simulink model "AGC30Model_ex1_11"  (R2021a)
settings: Solver=ode4  StartTime=stime  StopTime=etime  FixedStep=dtload  RelTol=1e-3
values from neighbouring files (symbols this model uses):
  AL_A = 0.3    [init_lfc_model.m]
  AL_B = 0.3    [init_lfc_model.m]
  DELTA_CC = Delta_cc_ty(TY_CC)    [load_thermal_constants.m]
  DELTA_ST = Delta_st_ty(TY_ST)    [load_thermal_constants.m]
  dtload = 0.1    [initset_dataload.m]
  F0 = 60    [init_inertia_model.m]    (also in initset_inertia.m)
  FFCS0_CC = (WF0_CC-WF_MIN_CC)./(1.0-WF_MIN_CC)    [calc_thermal_init_values.m]    (also in init_thermals.m)
  FGT_CC = Fgt_cc_ty(TY_CC)    [load_thermal_constants.m]
  FX_FB_CC = Fx_fb_cc_ty(:,TY_CC)    [load_thermal_constants.m]
  FX_FB_ST = Fx_fb_st_ty(:,TY_ST)    [load_thermal_constants.m]
  FX_FB_WT = FX_FB_WT_ty(:,TY_WT)    [load_const_hydro_constants.m]
  FX_N_GN_VA = FX_N_GN_VA_ty(:,TY_VA)    [load_var_hydro_constants.m]
  FX_N_PM_VA = FX_N_PM_VA_ty(:,TY_VA)    [load_var_hydro_constants.m]
  FX_PTHD_ST = Fx_pthd_st_ty(:,TY_ST)    [load_thermal_constants.m]
  FX_T_PM_VA = FX_T_PM_VA_ty(:,TY_VA)    [load_var_hydro_constants.m]
  FX_TE1_CC = Fx_te1_cc_ty(:,TY_CC)    [load_thermal_constants.m]
  FX_TE2_CC = Fx_te2_cc_ty(:,TY_CC)    [load_thermal_constants.m]
  FX_Y_GN_VA = FX_Y_GN_VA_ty(:,TY_VA)    [load_var_hydro_constants.m]
  FX_Y_PM_VA = FX_Y_PM_VA_ty(:,TY_VA)    [load_var_hydro_constants.m]
  FY_FB_CC = Fy_fb_cc_ty(:,TY_CC)    [load_thermal_constants.m]
  FY_FB_ST = Fy_fb_st_ty(:,TY_ST)    [load_thermal_constants.m]
  FY_FB_WT = FY_FB_WT_ty(:,TY_WT)    [load_const_hydro_constants.m]
  FY_N_GN_VA = FY_N_GN_VA_ty(:,TY_VA)    [load_var_hydro_constants.m]
  FY_N_PM_VA = FY_N_PM_VA_ty(:,TY_VA)    [load_var_hydro_constants.m]
  FY_PTHD_ST = Fy_pthd_st_ty(:,TY_ST)    [load_thermal_constants.m]
  FY_T_PM_VA = FY_T_PM_VA_ty(:,TY_VA)    [load_var_hydro_constants.m]
  FY_TE1_CC = Fy_te1_cc_ty(:,TY_CC)    [load_thermal_constants.m]
  FY_TE2_CC = Fy_te2_cc_ty(:,TY_CC)    [load_thermal_constants.m]
  FY_Y_GN_VA = FY_Y_GN_VA_ty(:,TY_VA)    [load_var_hydro_constants.m]
  FY_Y_PM_VA = FY_Y_PM_VA_ty(:,TY_VA)    [load_var_hydro_constants.m]
  G_cost = [Cost(:,3) ... (first row only)    [initset_dataload.m]
  G_down_limit = max(G_down_limit, G_out_pre - G_speed*5)    [calc_edc_output.m]    (also in edc.m; initset_dataload.m = csvread('G_down_plan_limit.csv',0,1))
  G_G_ST = G_g_st_ty(TY_ST)    [load_thermal_constants.m]
  G_speed = u(220:249,1)    [calc_edc_output.m]    (also in edc.m; initset_dataload.m = G_speed(:,1))
  GF_CC = [1, 1, 1, 1, 1,            1, 1, 1, 1, 1]    [init_thermal_model.m]
  GF_ST = [1, 1, 1, 1, 1, 1, 1,            1, 1, 1, 1,            1, 1, 1, 1, 1, 1]    [init_thermal_model.m]
  GMW_CC = Gmw_cc_ty(TY_CC)    [load_thermal_constants.m]
  GMW_ST = Gmw_st_ty(TY_ST)    [load_thermal_constants.m]
  GMW_VA = GMW_VA_ty(TY_VA)    [load_var_hydro_constants.m]
  GMW_WT = GMW_WT_ty(TY_WT)    [load_const_hydro_constants.m]
  HC_CC = Hc_cc_ty(TY_CC)    [load_thermal_constants.m]
  HT_CC = Ht_cc_ty(TY_CC)    [load_thermal_constants.m]
  IGV0_CC = WF0_CC    [calc_thermal_init_values.m]    (also in init_thermals.m)
  inertia_input = inertia_input'    [initset_dataload.m]
  K1_CONV_VA = K1_CONV_VA_ty(TY_VA)    [load_var_hydro_constants.m]
  K1_CONV_WT = K1_CONV_WT_ty(TY_WT)    [load_const_hydro_constants.m]
  K2_SERV_VA = K2_SERV_VA_ty(TY_VA)    [load_var_hydro_constants.m]
  K2_SERV_WT = K2_SERV_WT_ty(TY_WT)    [load_const_hydro_constants.m]
  K_A = 0.1    [init_lfc_model.m]
  K_B = 0.1    [init_lfc_model.m]
  K_G_ST = K_g_st_ty(TY_ST)    [load_thermal_constants.m]
  K_IGV_CC = K_igv_cc_ty(TY_CC)    [load_thermal_constants.m]
  K_L = 2.0    (= 2)    [init_inertia_model.m]    (also in initset_inertia.m)
  K_MW_GV_VA = K_MW_GV_VA_ty(TY_VA)    [load_var_hydro_constants.m]
  K_PREF_ST = K_pref_st_ty(TY_ST)    [load_thermal_constants.m]
  K_SD_VA = K_SD_VA_ty(TY_VA)    [load_var_hydro_constants.m]
  K_SD_WT = K_SD_WT_ty(TY_WT)    [load_const_hydro_constants.m]
  K_SEQ_WT = K_SEQ_WT_ty(TY_WT)    [load_const_hydro_constants.m]
  K_TE_CC = K_te_cc_ty(TY_CC)    [load_thermal_constants.m]
  KD_PID_VA = KD_PID_VA_ty(TY_VA)    [load_var_hydro_constants.m]
  KD_PID_WT = KD_PID_WT_ty(TY_WT)    [load_const_hydro_constants.m]
  KD_SG_GN_VA = KD_SG_GN_VA_ty(TY_VA)    [load_var_hydro_constants.m]
  KD_SG_PM_VA = KD_SG_PM_VA_ty(TY_VA)    [load_var_hydro_constants.m]
  KGT_CC = FGT_CC./((TFR_CC-TER_CC)-(TDR_CC-TIR_CC))    [calc_thermal_init_values.m]    (also in init_thermals.m)
  KI_PID_VA = KI_PID_VA_ty(TY_VA)    [load_var_hydro_constants.m]
  KI_PID_WT = KI_PID_WT_ty(TY_WT)    [load_const_hydro_constants.m]
  KI_SG_GN_VA = KI_SG_GN_VA_ty(TY_VA)    [load_var_hydro_constants.m]
  KI_SG_PM_VA = KI_SG_PM_VA_ty(TY_VA)    [load_var_hydro_constants.m]
  KP_A = 1.0    (= 1)    [init_lfc_model.m]
  KP_B = 1.0    (= 1)    [init_lfc_model.m]
  KP_PID_VA = KP_PID_VA_ty(TY_VA)    [load_var_hydro_constants.m]
  KP_PID_WT = KP_PID_WT_ty(TY_WT)    [load_const_hydro_constants.m]
  KP_SG_GN_VA = KP_SG_GN_VA_ty(TY_VA)    [load_var_hydro_constants.m]
  KP_SG_PM_VA = KP_SG_PM_VA_ty(TY_VA)    [load_var_hydro_constants.m]
  KST_CC = (1.0-FGT_CC)./TER_CC    [calc_thermal_init_values.m]    (also in init_thermals.m)
  L_FUEL_CC = L_fuel_cc_ty(TY_CC)    [load_thermal_constants.m]
  L_G_ST = L_g_st_ty(TY_ST)    [load_thermal_constants.m]
  L_IGV_CC = L_igv_cc_ty(TY_CC)    [load_thermal_constants.m]
  L_LL_ST = L_ll_st_ty(TY_ST)    [load_thermal_constants.m]
  L_MWD_CC = L_mwd_cc_ty(TY_CC)    [load_thermal_constants.m]
  L_MWD_GN_VA = L_MWD_GN_VA_ty(TY_VA)    [load_var_hydro_constants.m]
  L_MWD_PM_VA = L_MWD_PM_VA_ty(TY_VA)    [load_var_hydro_constants.m]
  L_MWD_ST = L_mwd_st_ty(TY_ST)    [load_thermal_constants.m]
  L_MWD_WT = L_MWD_WT_ty(TY_WT)    [load_const_hydro_constants.m]
  L_PREF_CC = L_pref_cc_ty(TY_CC)    [load_thermal_constants.m]
  L_PREF_ST = L_pref_st_ty(TY_ST)    [load_thermal_constants.m]
  LFC_cycle = 5.0    (= 5)    [init_lfc_model.m]
  load_input = load_input(:,stime+1:etime+1)    [initset_dataload.m]
  M_VA = M_VA_ty(TY_VA)    [load_var_hydro_constants.m]
  MVABase = 1000    [init_inertia_model.m]    (also in initset_inertia.m)
  MW0_ST = zeros(1,17)    [calc_thermal_init_values.m]    (also in init_thermals.m)
  MW0_WT = zeros(1,2)    [calc_const_hydro_init_values.m]    (also in init_conhydros.m)
  P_G_CONV_WT = P_G_CONV_WT_ty(TY_WT)    [load_const_hydro_constants.m]
  PG_INIT_CC = PMWD_SCHEDULE(1,19:28)'    [calc_thermal_init_values.m]    (also in init_thermals.m)
  PLM_CC = Plm_cc_ty(TY_CC)    [load_thermal_constants.m]
  PLM_ST = Plm_st_ty(TY_ST)    [load_thermal_constants.m]
  PMAX_B = 360.0    (= 360)    [init_lfc_model.m]
  PMIN_B = -360.0    (= -360)    [init_lfc_model.m]
  PMST0_CC = zeros(1, 10)    [calc_thermal_init_values.m]    (also in init_thermals.m)
  PMWD_EDC0 = zeros(1,30)    [init_edc_model.m]    (also in initset_edc.m)
  PMWD_SCHEDULE = u(3:32,1)    [calc_edc_output.m]    (also in edc.m; init_edc_model.m = g_out_input'; initset_edc.m = g_out_input')
  PRC_CC = Prc_cc_ty(TY_CC)    [load_thermal_constants.m]
  PRT_CC = PRC_CC.*(1-EP_CC)    [calc_thermal_init_values.m]    (also in init_thermals.m)
  PTH0_ST = zeros(1,17)    [calc_thermal_init_values.m]    (also in init_thermals.m)
  R_LL_ST = R_ll_st_ty(TY_ST)    [load_thermal_constants.m]
  R_MWD_CC = R_mwd_cc_ty(TY_CC)    [load_thermal_constants.m]
  R_MWD_ST = R_mwd_st_ty(TY_ST)    [load_thermal_constants.m]
  R_PREF_CC = R_pref_cc_ty(TY_CC)    [load_thermal_constants.m]
  RA_A = G_speed'    [init_lfc_model.m]
  RA_B = 96.0    (= 96)    [init_lfc_model.m]
  RATE_GN_VA = RATE_GN_VA_ty(TY_VA)    [load_var_hydro_constants.m]
  RATE_PM_VA = RATE_PM_VA_ty(TY_VA)    [load_var_hydro_constants.m]
  RC_CC = Rc_cc_ty(TY_CC)    [load_thermal_constants.m]
  RT_CC = Rt_cc_ty(TY_CC)    [load_thermal_constants.m]
  SW_T_ST = Sw_t_st_ty(TY_ST)    [load_thermal_constants.m]
  T1_B_ST = T1_b_st_ty(TY_ST)    [load_thermal_constants.m]
  T1_CONV_VA = T1_CONV_VA_ty(TY_VA)    [load_var_hydro_constants.m]
  T1_CONV_WT = T1_CONV_WT_ty(TY_WT)    [load_const_hydro_constants.m]
  T1_G_ST = T1_g_st_ty(TY_ST)    [load_thermal_constants.m]
  T2_B_ST = T2_b_st_ty(TY_ST)    [load_thermal_constants.m]
  ... (+53 more)
undefined symbols (not defined in the file or in its folder): DELTA_B, DiscIntNeverNeededParam, FX_FB_ST_OA, FX_PTHD_ST_OA, FY_FB_ST_OA, FY_PTHD_ST_OA, G_G_ST_OA, K_G_ST_OA, K_PREF_ST_OA, MW0_ST_OA, N_GN_INIT_VA, N_PM_INIT_VA, PLM_B, R_LL_ST_OA, T1_B_ST_OA, T1_G_ST_OA, T2_B_ST_OA, T2_G_ST_OA, T3_B_ST_OA, T4_G_ST_OA, T5_G_ST_OA, T_LL_ST_OA, T_PREF_ST_OA, Y_GN_INIT_VA, Y_PM_INIT_VA
libraries: simulink_extras x87, simulink x42, pid_lib x1
(part 3 of 5)

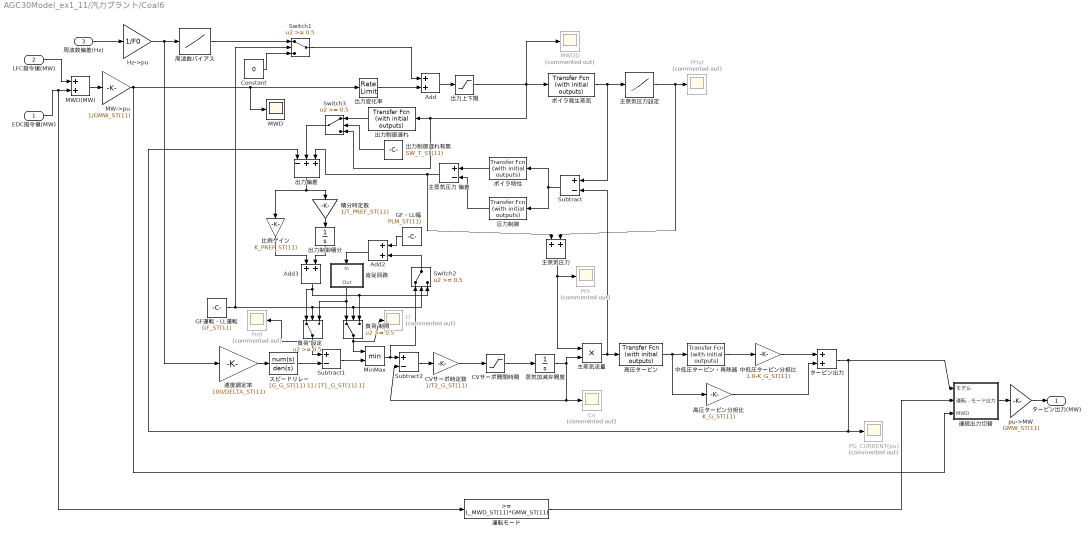
== system AGC30Model_ex1_11/汽力プラント/Coal6 ==
  EDC指令値(MW) : Inport
  LFC指令値(MW) : Inport  Port=2
  周波数偏差(Hz) : Inport  Port=3
  Add : Sum
  Add2 : Sum
  Add3 : Sum
  CVサーボ時定数 : Gain  Gain=1/T2_G_ST(11)
  CVサーボ開閉時間 : Saturate  UpperLimit=1/T3_G_ST(11)  LowerLimit=1/T6_G_ST(11)
  Constant : Constant  Value=0
  Cv : Scope  Commented=on
  GF・LL幅 : Constant  Value=PLM_ST(11)
  GF運転・LL運転 : Constant  Value=GF_ST(11)
  Hz->pu : Gain  Gain=1/F0
  Ll : Scope  Commented=on
  MW->pu : Gain  Gain=1/GMW_ST(11)
  MWD : Scope
  MWD(MW) : Sum
  MWDD : Scope  Commented=on
  MinMax : MinMax  Inputs=2
  PG_CURRENT(pu) : Scope  Commented=on
  Pref : Scope  Commented=on
  Pth : Scope  Commented=on
  Pthd : Scope  Commented=on
  Subtract : Sum  Inputs=+-
  Subtract1 : Sum  Inputs=+-
  Subtract2 : Sum  Inputs=+-
  Switch1 : Switch  Threshold=0.5
  Switch2 : Switch  Threshold=0.5
  Switch3 : Switch  Threshold=0.5
  pu->MW : Gain  Gain=GMW_ST(11)
  スピードリレー : TransferFcn  Numerator=[G_G_ST(11) 1]  Denominator=[T1_G_ST(11) 1]
  タービン出力 : Sum
  ボイラ特性 : simulink_extras/Additional Linear/Transfer Fcn (with initial outputs)  N=[1]  D=[T2_B_ST(11) 1]  Y0=0  U0=0
  ボイラ発生蒸気 : simulink_extras/Additional Linear/Transfer Fcn (with initial outputs)  N=[1]  D=[T1_B_ST(11) 1]  Y0=MW0_ST(11)  U0=MW0_ST(11)
  中低圧タービン・再熱器 : simulink_extras/Additional Linear/Transfer Fcn (with initial outputs)  N=[1]  D=[T5_G_ST(11) 1]  Y0=MW0_ST(11)  U0=MW0_ST(11)
  中低圧タービン分担比 : Gain  Gain=1.0-K_G_ST(11)
  主蒸気圧力 : Sum
  主蒸気圧力 偏差 : Sum  Inputs=+-
  主蒸気圧力設定 : Lookup  InputValues=FX_PTHD_ST(:,11)  Table=FY_PTHD_ST(:,11)  LookUpMeth=Interpolation-Use End Values
  主蒸気流量 : Product  RndMeth=Zero
  出力上下限 : Saturate  UpperLimit=U_MWD_ST(11)  LowerLimit=L_MWD_ST(11)
  出力偏差 : Sum  Inputs=-++
  出力制御積分 : Integrator  InitialCondition=MW0_ST(11)/PTH0_ST(11)  LimitOutput=on  UpperSaturationLimit=U_PREF_ST(11)  LowerSaturationLimit=L_PREF_ST(11)
  出力制御遅れ : simulink_extras/Additional Linear/Transfer Fcn (with initial outputs)  N=[1]  D=[T_T_ST(11) 1]  Y0=MW0_ST(11)  U0=MW0_ST(11)
  出力制御遅れ有無 : Constant  Value=SW_T_ST(11)
  出力変化率 : RateLimiter  RisingSlewLimit=R_MWD_ST(11)/60  FallingSlewLimit=-R_MWD_ST(11)/60  SampleTimeMode=inherited  InitialCondition=MW0_ST(11)
  周波数バイアス : Lookup  InputValues=FX_FB_ST(:,11)/F0  Table=FY_FB_ST(:,11)  LookUpMeth=Interpolation-Use End Values
  圧力制御 : simulink_extras/Additional Linear/Transfer Fcn (with initial outputs)  N=[1]  D=[T3_B_ST(11) 1]  Y0=0  U0=0
  比例ゲイン : Gain  Gain=K_PREF_ST(11)
  積分時定数 : Gain  Gain=1/T_PREF_ST(11)
  蒸気加減弁開度 : Integrator  InitialCondition=MW0_ST(11)/PTH0_ST(11)  LimitOutput=on  UpperSaturationLimit=U_G_ST(11)  LowerSaturationLimit=L_G_ST(11)
  負荷 制限 : Switch  Threshold=0.5
  負荷 設定 : Switch  Threshold=0.5
  追従回路 : Subsystem
  速度調定率 : Gain  Gain=100/DELTA_ST(11)
  連続出力切替 : Subsystem
  運転モード : simulink/Logic and Bit Operations/Compare To Constant  relop=>=  const=L_MWD_ST(11)*GMW_ST(11)  OutDataTypeStr=boolean
  高圧タービン : simulink_extras/Additional Linear/Transfer Fcn (with initial outputs)  N=[1]  D=[T4_G_ST(11) 1]  Y0=MW0_ST(11)  U0=MW0_ST(11)
  高圧タービン分担比 : Gain  Gain=K_G_ST(11)
  タービン出力(MW) : Outport  VectorParamsAs1DForOutWhenUnconnected=off
  wires:
  MWD(MW)/1 -> MW->pu/1
  周波数偏差(Hz)/1 -> Hz->pu/1
  Add/1 -> 出力上下限/1
  出力変化率/1 -> Add/2
  ボイラ発生蒸気/1 -> Subtract/1, 主蒸気圧力設定/1
  出力偏差/1 -> 比例ゲイン/1, 積分時定数/1
  比例ゲイン/1 -> Add3/1
  Add3/1 -> 負荷 制限/3, Switch2/3, 負荷 設定/1
  主蒸気圧力 偏差/1 -> 主蒸気圧力/1, 出力偏差/3
  主蒸気圧力設定/1 -> Pthd/1, 主蒸気圧力/2
  主蒸気流量/1 -> Subtract/2, 高圧タービン/1
  積分時定数/1 -> 出力制御積分/1
  出力制御積分/1 -> Add3/2
  速度調定率/1 -> スピードリレー/1
  Subtract1/1 -> MinMax/2
  主蒸気圧力/1 -> 主蒸気流量/1, Pth/1
  スピードリレー/1 -> Subtract1/2
  MinMax/1 -> Subtract2/1, Switch2/1
  Subtract2/1 -> CVサーボ時定数/1
  CVサーボ時定数/1 -> CVサーボ開閉時間/1
  CVサーボ開閉時間/1 -> 蒸気加減弁開度/1
  蒸気加減弁開度/1 -> 主蒸気流量/2, Subtract2/2, Cv/1
  高圧タービン/1 -> 中低圧タービン・再熱器/1, 高圧タービン分担比/1
  中低圧タービン・再熱器/1 -> 中低圧タービン分担比/1
  高圧タービン分担比/1 -> タービン出力/2
  中低圧タービン分担比/1 -> タービン出力/1
  タービン出力/1 -> 出力偏差/1, PG_CURRENT(pu)/1, 連続出力切替/1(モデル)
  GF・LL幅/1 -> Add2/1
  Add2/1 -> 追従回路/1(In)
  ボイラ特性/1 -> 主蒸気圧力 偏差/1
  圧力制御/1 -> 主蒸気圧力 偏差/2
  Subtract/1 -> ボイラ特性/1, 圧力制御/1
  出力上下限/1 -> ボイラ発生蒸気/1, MWDD/1, 出力制御遅れ/1, Switch3/3
  GF運転・LL運転/1 -> 負荷 設定/2, 負荷 制限/2, Switch2/2, Switch1/2
  負荷 設定/1 -> Subtract1/1, Pref/1
  追従回路/1(Out) -> 負荷 制限/1, 負荷 設定/3
  Switch2/1 -> Add2/2
  MW->pu/1 -> MWD/1, 出力変化率/1, 連続出力切替/3(MWD)
  Hz->pu/1 -> 速度調定率/1, 周波数バイアス/1
  連続出力切替/1(出力) -> pu->MW/1
  pu->MW/1 -> タービン出力(MW)/1
  負荷 制限/1 -> MinMax/1, Ll/1
  周波数バイアス/1 -> Switch1/1
  Constant/1 -> Switch1/3
  Switch1/1 -> Add/1
  出力制御遅れ/1 -> Switch3/1
  Switch3/1 -> 出力偏差/2
  出力制御遅れ有無/1 -> Switch3/2
  EDC指令値(MW)/1 -> MWD(MW)/2, 運転モード/1
  LFC指令値(MW)/1 -> MWD(MW)/1
  運転モード/1 -> 連続出力切替/2(運転モード)

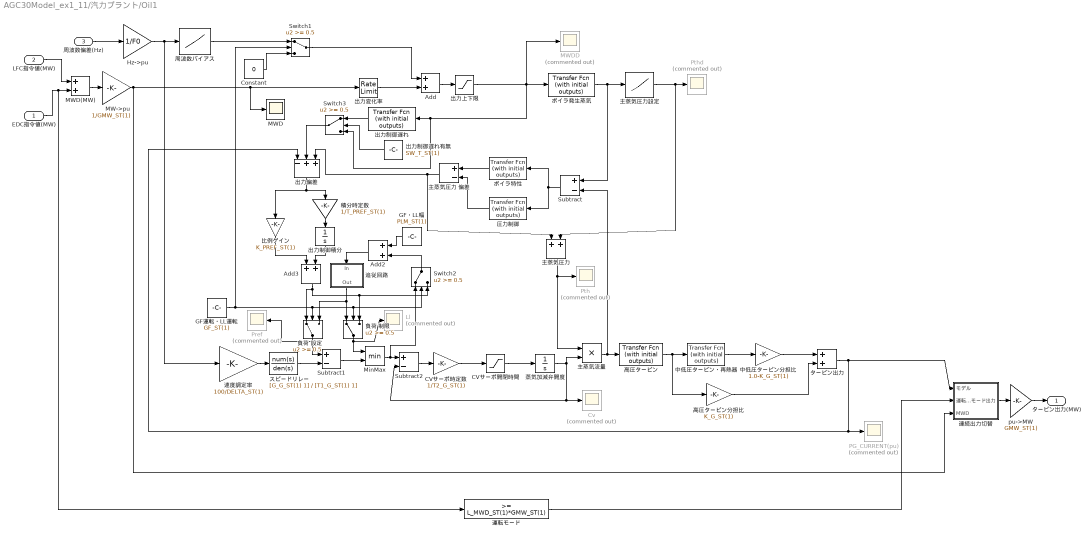
== system AGC30Model_ex1_11/汽力プラント/Oil1 ==
  EDC指令値(MW) : Inport
  LFC指令値(MW) : Inport  Port=2
  周波数偏差(Hz) : Inport  Port=3
  Add : Sum
  Add2 : Sum
  Add3 : Sum
  CVサーボ時定数 : Gain  Gain=1/T2_G_ST(1)
  CVサーボ開閉時間 : Saturate  UpperLimit=1/T3_G_ST(1)  LowerLimit=1/T6_G_ST(1)
  Constant : Constant  Value=0
  Cv : Scope  Commented=on
  GF・LL幅 : Constant  Value=PLM_ST(1)
  GF運転・LL運転 : Constant  Value=GF_ST(1)
  Hz->pu : Gain  Gain=1/F0
  Ll : Scope  Commented=on
  MW->pu : Gain  Gain=1/GMW_ST(1)
  MWD : Scope
  MWD(MW) : Sum
  MWDD : Scope  Commented=on
  MinMax : MinMax  Inputs=2
  PG_CURRENT(pu) : Scope  Commented=on
  Pref : Scope  Commented=on
  Pth : Scope  Commented=on
  Pthd : Scope  Commented=on
  Subtract : Sum  Inputs=+-
  Subtract1 : Sum  Inputs=+-
  Subtract2 : Sum  Inputs=+-
  Switch1 : Switch  Threshold=0.5
  Switch2 : Switch  Threshold=0.5
  Switch3 : Switch  Threshold=0.5
  pu->MW : Gain  Gain=GMW_ST(1)
  スピードリレー : TransferFcn  Numerator=[G_G_ST(1) 1]  Denominator=[T1_G_ST(1) 1]
  タービン出力 : Sum
  ボイラ特性 : simulink_extras/Additional Linear/Transfer Fcn (with initial outputs)  N=[1]  D=[T2_B_ST(1) 1]  Y0=0  U0=0
  ボイラ発生蒸気 : simulink_extras/Additional Linear/Transfer Fcn (with initial outputs)  N=[1]  D=[T1_B_ST(1) 1]  Y0=MW0_ST(1)  U0=MW0_ST(1)
  中低圧タービン・再熱器 : simulink_extras/Additional Linear/Transfer Fcn (with initial outputs)  N=[1]  D=[T5_G_ST(1) 1]  Y0=MW0_ST(1)  U0=MW0_ST(1)
  中低圧タービン分担比 : Gain  Gain=1.0-K_G_ST(1)
  主蒸気圧力 : Sum
  主蒸気圧力 偏差 : Sum  Inputs=+-
  主蒸気圧力設定 : Lookup  InputValues=FX_PTHD_ST(:,1)  Table=FY_PTHD_ST(:,1)  LookUpMeth=Interpolation-Use End Values
  主蒸気流量 : Product  RndMeth=Zero
  出力上下限 : Saturate  UpperLimit=U_MWD_ST(1)  LowerLimit=L_MWD_ST(1)
  出力偏差 : Sum  Inputs=-++
  出力制御積分 : Integrator  InitialCondition=MW0_ST(1)/PTH0_ST(1)  LimitOutput=on  UpperSaturationLimit=U_PREF_ST(1)  LowerSaturationLimit=L_PREF_ST(1)
  出力制御遅れ : simulink_extras/Additional Linear/Transfer Fcn (with initial outputs)  N=[1]  D=[T_T_ST(1) 1]  Y0=MW0_ST(1)  U0=MW0_ST(1)
  出力制御遅れ有無 : Constant  Value=SW_T_ST(1)
  出力変化率 : RateLimiter  RisingSlewLimit=R_MWD_ST(1)/60  FallingSlewLimit=-R_MWD_ST(1)/60  SampleTimeMode=inherited  InitialCondition=MW0_ST(1)
  周波数バイアス : Lookup  InputValues=FX_FB_ST(:,1)/F0  Table=FY_FB_ST(:,1)  LookUpMeth=Interpolation-Use End Values
  圧力制御 : simulink_extras/Additional Linear/Transfer Fcn (with initial outputs)  N=[1]  D=[T3_B_ST(1) 1]  Y0=0  U0=0
  比例ゲイン : Gain  Gain=K_PREF_ST(1)
  積分時定数 : Gain  Gain=1/T_PREF_ST(1)
  蒸気加減弁開度 : Integrator  InitialCondition=MW0_ST(1)/PTH0_ST(1)  LimitOutput=on  UpperSaturationLimit=U_G_ST(1)  LowerSaturationLimit=L_G_ST(1)
  負荷 制限 : Switch  Threshold=0.5
  負荷 設定 : Switch  Threshold=0.5
  追従回路 : Subsystem
  速度調定率 : Gain  Gain=100/DELTA_ST(1)
  連続出力切替 : Subsystem
  運転モード : simulink/Logic and Bit Operations/Compare To Constant  relop=>=  const=L_MWD_ST(1)*GMW_ST(1)  OutDataTypeStr=boolean
  高圧タービン : simulink_extras/Additional Linear/Transfer Fcn (with initial outputs)  N=[1]  D=[T4_G_ST(1) 1]  Y0=MW0_ST(1)  U0=MW0_ST(1)
  高圧タービン分担比 : Gain  Gain=K_G_ST(1)
  タービン出力(MW) : Outport  VectorParamsAs1DForOutWhenUnconnected=off
  wires:
  MWD(MW)/1 -> MW->pu/1
  周波数偏差(Hz)/1 -> Hz->pu/1
  Add/1 -> 出力上下限/1
  出力変化率/1 -> Add/2
  ボイラ発生蒸気/1 -> Subtract/1, 主蒸気圧力設定/1
  出力偏差/1 -> 比例ゲイン/1, 積分時定数/1
  比例ゲイン/1 -> Add3/1
  Add3/1 -> 負荷 制限/3, Switch2/3, 負荷 設定/1
  主蒸気圧力 偏差/1 -> 主蒸気圧力/1, 出力偏差/3
  主蒸気圧力設定/1 -> Pthd/1, 主蒸気圧力/2
  主蒸気流量/1 -> Subtract/2, 高圧タービン/1
  積分時定数/1 -> 出力制御積分/1
  出力制御積分/1 -> Add3/2
  速度調定率/1 -> スピードリレー/1
  Subtract1/1 -> MinMax/2
  主蒸気圧力/1 -> 主蒸気流量/1, Pth/1
  スピードリレー/1 -> Subtract1/2
  MinMax/1 -> Subtract2/1, Switch2/1
  Subtract2/1 -> CVサーボ時定数/1
  CVサーボ時定数/1 -> CVサーボ開閉時間/1
  CVサーボ開閉時間/1 -> 蒸気加減弁開度/1
  蒸気加減弁開度/1 -> 主蒸気流量/2, Subtract2/2, Cv/1
  高圧タービン/1 -> 中低圧タービン・再熱器/1, 高圧タービン分担比/1
  中低圧タービン・再熱器/1 -> 中低圧タービン分担比/1
  高圧タービン分担比/1 -> タービン出力/2
  中低圧タービン分担比/1 -> タービン出力/1
  タービン出力/1 -> 出力偏差/1, PG_CURRENT(pu)/1, 連続出力切替/1(モデル)
  GF・LL幅/1 -> Add2/1
  Add2/1 -> 追従回路/1(In)
  ボイラ特性/1 -> 主蒸気圧力 偏差/1
  圧力制御/1 -> 主蒸気圧力 偏差/2
  Subtract/1 -> ボイラ特性/1, 圧力制御/1
  出力上下限/1 -> ボイラ発生蒸気/1, MWDD/1, 出力制御遅れ/1, Switch3/3
  GF運転・LL運転/1 -> 負荷 設定/2, 負荷 制限/2, Switch2/2, Switch1/2
  負荷 設定/1 -> Subtract1/1, Pref/1
  追従回路/1(Out) -> 負荷 制限/1, 負荷 設定/3
  Switch2/1 -> Add2/2
  MW->pu/1 -> MWD/1, 出力変化率/1, 連続出力切替/3(MWD)
  Hz->pu/1 -> 速度調定率/1, 周波数バイアス/1
  連続出力切替/1(出力) -> pu->MW/1
  pu->MW/1 -> タービン出力(MW)/1
  負荷 制限/1 -> MinMax/1, Ll/1
  周波数バイアス/1 -> Switch1/1
  Constant/1 -> Switch1/3
  Switch1/1 -> Add/1
  出力制御遅れ/1 -> Switch3/1
  Switch3/1 -> 出力偏差/2
  出力制御遅れ有無/1 -> Switch3/2
  EDC指令値(MW)/1 -> MWD(MW)/2, 運転モード/1
  LFC指令値(MW)/1 -> MWD(MW)/1
  運転モード/1 -> 連続出力切替/2(運転モード)

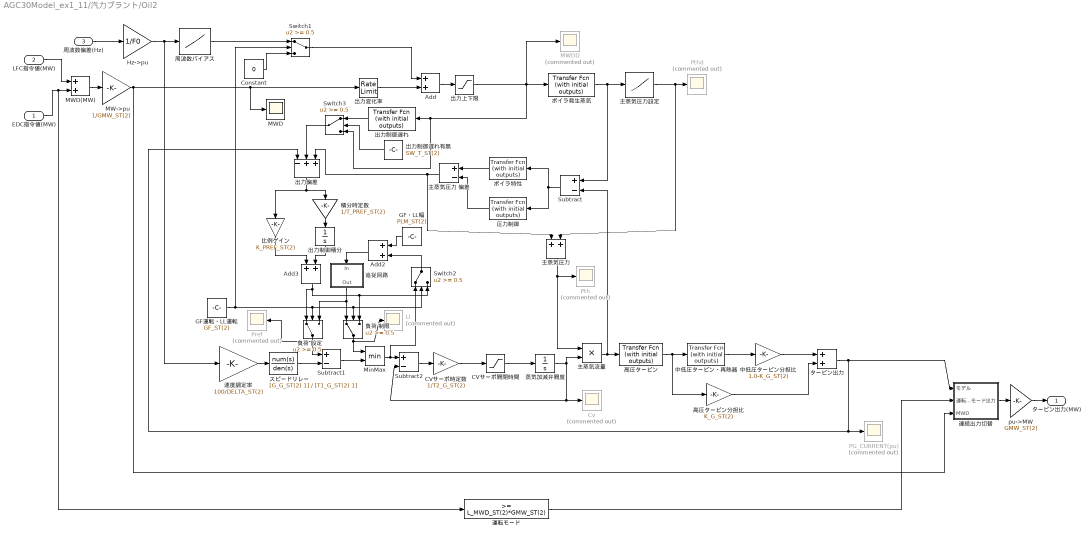
== system AGC30Model_ex1_11/汽力プラント/Oil2 ==
  EDC指令値(MW) : Inport
  LFC指令値(MW) : Inport  Port=2
  周波数偏差(Hz) : Inport  Port=3
  Add : Sum
  Add2 : Sum
  Add3 : Sum
  CVサーボ時定数 : Gain  Gain=1/T2_G_ST(2)
  CVサーボ開閉時間 : Saturate  UpperLimit=1/T3_G_ST(2)  LowerLimit=1/T6_G_ST(2)
  Constant : Constant  Value=0
  Cv : Scope  Commented=on
  GF・LL幅 : Constant  Value=PLM_ST(2)
  GF運転・LL運転 : Constant  Value=GF_ST(2)
  Hz->pu : Gain  Gain=1/F0
  Ll : Scope  Commented=on
  MW->pu : Gain  Gain=1/GMW_ST(2)
  MWD : Scope
  MWD(MW) : Sum
  MWDD : Scope  Commented=on
  MinMax : MinMax  Inputs=2
  PG_CURRENT(pu) : Scope  Commented=on
  Pref : Scope  Commented=on
  Pth : Scope  Commented=on
  Pthd : Scope  Commented=on
  Subtract : Sum  Inputs=+-
  Subtract1 : Sum  Inputs=+-
  Subtract2 : Sum  Inputs=+-
  Switch1 : Switch  Threshold=0.5
  Switch2 : Switch  Threshold=0.5
  Switch3 : Switch  Threshold=0.5
  pu->MW : Gain  Gain=GMW_ST(2)
  スピードリレー : TransferFcn  Numerator=[G_G_ST(2) 1]  Denominator=[T1_G_ST(2) 1]
  タービン出力 : Sum
  ボイラ特性 : simulink_extras/Additional Linear/Transfer Fcn (with initial outputs)  N=[1]  D=[T2_B_ST(2) 1]  Y0=0  U0=0
  ボイラ発生蒸気 : simulink_extras/Additional Linear/Transfer Fcn (with initial outputs)  N=[1]  D=[T1_B_ST(2) 1]  Y0=MW0_ST(2)  U0=MW0_ST(2)
  中低圧タービン・再熱器 : simulink_extras/Additional Linear/Transfer Fcn (with initial outputs)  N=[1]  D=[T5_G_ST(2) 1]  Y0=MW0_ST(2)  U0=MW0_ST(2)
  中低圧タービン分担比 : Gain  Gain=1.0-K_G_ST(2)
  主蒸気圧力 : Sum
  主蒸気圧力 偏差 : Sum  Inputs=+-
  主蒸気圧力設定 : Lookup  InputValues=FX_PTHD_ST(:,2)  Table=FY_PTHD_ST(:,2)  LookUpMeth=Interpolation-Use End Values
  主蒸気流量 : Product  RndMeth=Zero
  出力上下限 : Saturate  UpperLimit=U_MWD_ST(2)  LowerLimit=L_MWD_ST(2)
  出力偏差 : Sum  Inputs=-++
  出力制御積分 : Integrator  InitialCondition=MW0_ST(2)/PTH0_ST(2)  LimitOutput=on  UpperSaturationLimit=U_PREF_ST(2)  LowerSaturationLimit=L_PREF_ST(2)
  出力制御遅れ : simulink_extras/Additional Linear/Transfer Fcn (with initial outputs)  N=[1]  D=[T_T_ST(2) 1]  Y0=MW0_ST(2)  U0=MW0_ST(2)
  出力制御遅れ有無 : Constant  Value=SW_T_ST(2)
  出力変化率 : RateLimiter  RisingSlewLimit=R_MWD_ST(2)/60  FallingSlewLimit=-R_MWD_ST(2)/60  SampleTimeMode=inherited  InitialCondition=MW0_ST(2)
  周波数バイアス : Lookup  InputValues=FX_FB_ST(:,2)/F0  Table=FY_FB_ST(:,2)  LookUpMeth=Interpolation-Use End Values
  圧力制御 : simulink_extras/Additional Linear/Transfer Fcn (with initial outputs)  N=[1]  D=[T3_B_ST(2) 1]  Y0=0  U0=0
  比例ゲイン : Gain  Gain=K_PREF_ST(2)
  積分時定数 : Gain  Gain=1/T_PREF_ST(2)
  蒸気加減弁開度 : Integrator  InitialCondition=MW0_ST(2)/PTH0_ST(2)  LimitOutput=on  UpperSaturationLimit=U_G_ST(2)  LowerSaturationLimit=L_G_ST(2)
  負荷 制限 : Switch  Threshold=0.5
  負荷 設定 : Switch  Threshold=0.5
  追従回路 : Subsystem
  速度調定率 : Gain  Gain=100/DELTA_ST(2)
  連続出力切替 : Subsystem
  運転モード : simulink/Logic and Bit Operations/Compare To Constant  relop=>=  const=L_MWD_ST(2)*GMW_ST(2)  OutDataTypeStr=boolean
  高圧タービン : simulink_extras/Additional Linear/Transfer Fcn (with initial outputs)  N=[1]  D=[T4_G_ST(2) 1]  Y0=MW0_ST(2)  U0=MW0_ST(2)
  高圧タービン分担比 : Gain  Gain=K_G_ST(2)
  タービン出力(MW) : Outport  VectorParamsAs1DForOutWhenUnconnected=off
  wires:
  MWD(MW)/1 -> MW->pu/1
  周波数偏差(Hz)/1 -> Hz->pu/1
  Add/1 -> 出力上下限/1
  出力変化率/1 -> Add/2
  ボイラ発生蒸気/1 -> Subtract/1, 主蒸気圧力設定/1
  出力偏差/1 -> 比例ゲイン/1, 積分時定数/1
  比例ゲイン/1 -> Add3/1
  Add3/1 -> 負荷 制限/3, Switch2/3, 負荷 設定/1
  主蒸気圧力 偏差/1 -> 主蒸気圧力/1, 出力偏差/3
  主蒸気圧力設定/1 -> Pthd/1, 主蒸気圧力/2
  主蒸気流量/1 -> Subtract/2, 高圧タービン/1
  積分時定数/1 -> 出力制御積分/1
  出力制御積分/1 -> Add3/2
  速度調定率/1 -> スピードリレー/1
  Subtract1/1 -> MinMax/2
  主蒸気圧力/1 -> 主蒸気流量/1, Pth/1
  スピードリレー/1 -> Subtract1/2
  MinMax/1 -> Subtract2/1, Switch2/1
  Subtract2/1 -> CVサーボ時定数/1
  CVサーボ時定数/1 -> CVサーボ開閉時間/1
  CVサーボ開閉時間/1 -> 蒸気加減弁開度/1
  蒸気加減弁開度/1 -> 主蒸気流量/2, Subtract2/2, Cv/1
  高圧タービン/1 -> 中低圧タービン・再熱器/1, 高圧タービン分担比/1
  中低圧タービン・再熱器/1 -> 中低圧タービン分担比/1
  高圧タービン分担比/1 -> タービン出力/2
  中低圧タービン分担比/1 -> タービン出力/1
  タービン出力/1 -> 出力偏差/1, PG_CURRENT(pu)/1, 連続出力切替/1(モデル)
  GF・LL幅/1 -> Add2/1
  Add2/1 -> 追従回路/1(In)
  ボイラ特性/1 -> 主蒸気圧力 偏差/1
  圧力制御/1 -> 主蒸気圧力 偏差/2
  Subtract/1 -> ボイラ特性/1, 圧力制御/1
  出力上下限/1 -> ボイラ発生蒸気/1, MWDD/1, 出力制御遅れ/1, Switch3/3
  GF運転・LL運転/1 -> 負荷 設定/2, 負荷 制限/2, Switch2/2, Switch1/2
  負荷 設定/1 -> Subtract1/1, Pref/1
  追従回路/1(Out) -> 負荷 制限/1, 負荷 設定/3
  Switch2/1 -> Add2/2
  MW->pu/1 -> MWD/1, 出力変化率/1, 連続出力切替/3(MWD)
  Hz->pu/1 -> 速度調定率/1, 周波数バイアス/1
  連続出力切替/1(出力) -> pu->MW/1
  pu->MW/1 -> タービン出力(MW)/1
  負荷 制限/1 -> MinMax/1, Ll/1
  周波数バイアス/1 -> Switch1/1
  Constant/1 -> Switch1/3
  Switch1/1 -> Add/1
  出力制御遅れ/1 -> Switch3/1
  Switch3/1 -> 出力偏差/2
  出力制御遅れ有無/1 -> Switch3/2
  EDC指令値(MW)/1 -> MWD(MW)/2, 運転モード/1
  LFC指令値(MW)/1 -> MWD(MW)/1
  運転モード/1 -> 連続出力切替/2(運転モード)

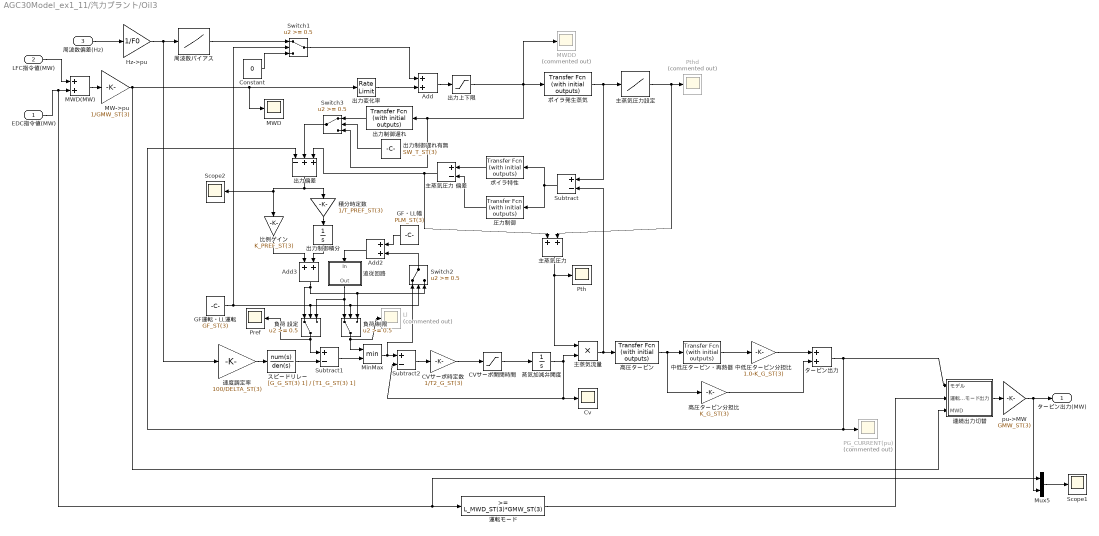
== system AGC30Model_ex1_11/汽力プラント/Oil3 ==
  EDC指令値(MW) : Inport
  LFC指令値(MW) : Inport  Port=2
  周波数偏差(Hz) : Inport  Port=3
  Add : Sum
  Add2 : Sum
  Add3 : Sum
  CVサーボ時定数 : Gain  Gain=1/T2_G_ST(3)
  CVサーボ開閉時間 : Saturate  UpperLimit=1/T3_G_ST(3)  LowerLimit=1/T6_G_ST(3)
  Constant : Constant  Value=0
  Cv : Scope
  GF・LL幅 : Constant  Value=PLM_ST(3)
  GF運転・LL運転 : Constant  Value=GF_ST(3)
  Hz->pu : Gain  Gain=1/F0
  Ll : Scope  Commented=on
  MW->pu : Gain  Gain=1/GMW_ST(3)
  MWD : Scope
  MWD(MW) : Sum
  MWDD : Scope  Commented=on
  MinMax : MinMax  Inputs=2
  Mux5 : Mux  Inputs=2
  PG_CURRENT(pu) : Scope  Commented=on
  Pref : Scope
  Pth : Scope
  Pthd : Scope  Commented=on
  Scope1 : Scope
  Scope2 : Scope
  Subtract : Sum  Inputs=+-
  Subtract1 : Sum  Inputs=+-
  Subtract2 : Sum  Inputs=+-
  Switch1 : Switch  Threshold=0.5
  Switch2 : Switch  Threshold=0.5
  Switch3 : Switch  Threshold=0.5
  pu->MW : Gain  Gain=GMW_ST(3)
  スピードリレー : TransferFcn  Numerator=[G_G_ST(3) 1]  Denominator=[T1_G_ST(3) 1]
  タービン出力 : Sum
  ボイラ特性 : simulink_extras/Additional Linear/Transfer Fcn (with initial outputs)  N=[1]  D=[T2_B_ST(3) 1]  Y0=0  U0=0
  ボイラ発生蒸気 : simulink_extras/Additional Linear/Transfer Fcn (with initial outputs)  N=[1]  D=[T1_B_ST(3) 1]  Y0=MW0_ST(3)  U0=MW0_ST(3)
  中低圧タービン・再熱器 : simulink_extras/Additional Linear/Transfer Fcn (with initial outputs)  N=[1]  D=[T5_G_ST(3) 1]  Y0=MW0_ST(3)  U0=MW0_ST(3)
  中低圧タービン分担比 : Gain  Gain=1.0-K_G_ST(3)
  主蒸気圧力 : Sum
  主蒸気圧力 偏差 : Sum  Inputs=+-
  主蒸気圧力設定 : Lookup  InputValues=FX_PTHD_ST(:,3)  Table=FY_PTHD_ST(:,3)  LookUpMeth=Interpolation-Use End Values
  主蒸気流量 : Product  RndMeth=Zero
  出力上下限 : Saturate  UpperLimit=U_MWD_ST(3)  LowerLimit=L_MWD_ST(3)
  出力偏差 : Sum  Inputs=-++
  出力制御積分 : Integrator  InitialCondition=MW0_ST(3)/PTH0_ST(3)  LimitOutput=on  UpperSaturationLimit=U_PREF_ST(3)  LowerSaturationLimit=L_PREF_ST(3)
  出力制御遅れ : simulink_extras/Additional Linear/Transfer Fcn (with initial outputs)  N=[1]  D=[T_T_ST(3) 1]  Y0=MW0_ST(3)  U0=MW0_ST(3)
  出力制御遅れ有無 : Constant  Value=SW_T_ST(3)
  出力変化率 : RateLimiter  RisingSlewLimit=R_MWD_ST(3)/60  FallingSlewLimit=-R_MWD_ST(3)/60  SampleTimeMode=inherited  InitialCondition=MW0_ST(3)
  周波数バイアス : Lookup  InputValues=FX_FB_ST(:,3)/F0  Table=FY_FB_ST(:,3)  LookUpMeth=Interpolation-Use End Values
  圧力制御 : simulink_extras/Additional Linear/Transfer Fcn (with initial outputs)  N=[1]  D=[T3_B_ST(3) 1]  Y0=0  U0=0
  比例ゲイン : Gain  Gain=K_PREF_ST(3)
  積分時定数 : Gain  Gain=1/T_PREF_ST(3)
  蒸気加減弁開度 : Integrator  InitialCondition=MW0_ST(3)/PTH0_ST(3)  LimitOutput=on  UpperSaturationLimit=U_G_ST(3)  LowerSaturationLimit=L_G_ST(3)
  負荷 制限 : Switch  Threshold=0.5
  負荷 設定 : Switch  Threshold=0.5
  追従回路 : Subsystem
  速度調定率 : Gain  Gain=100/DELTA_ST(3)
  連続出力切替 : Subsystem
  運転モード : simulink/Logic and Bit Operations/Compare To Constant  relop=>=  const=L_MWD_ST(3)*GMW_ST(3)  OutDataTypeStr=boolean
  高圧タービン : simulink_extras/Additional Linear/Transfer Fcn (with initial outputs)  N=[1]  D=[T4_G_ST(3) 1]  Y0=MW0_ST(3)  U0=MW0_ST(3)
  高圧タービン分担比 : Gain  Gain=K_G_ST(3)
  タービン出力(MW) : Outport  VectorParamsAs1DForOutWhenUnconnected=off
  wires:
  MWD(MW)/1 -> MW->pu/1
  周波数偏差(Hz)/1 -> Hz->pu/1
  Add/1 -> 出力上下限/1
  出力変化率/1 -> Add/2
  ボイラ発生蒸気/1 -> Subtract/1, 主蒸気圧力設定/1
  出力偏差/1 -> Scope2/1, 比例ゲイン/1, 積分時定数/1
  比例ゲイン/1 -> Add3/1
  Add3/1 -> 負荷 制限/3, Switch2/3, 負荷 設定/1
  主蒸気圧力 偏差/1 -> 主蒸気圧力/1, 出力偏差/3
  主蒸気圧力設定/1 -> Pthd/1, 主蒸気圧力/2
  主蒸気流量/1 -> Subtract/2, 高圧タービン/1
  積分時定数/1 -> 出力制御積分/1
  出力制御積分/1 -> Add3/2
  速度調定率/1 -> スピードリレー/1
  Subtract1/1 -> MinMax/2
  主蒸気圧力/1 -> 主蒸気流量/1, Pth/1
  スピードリレー/1 -> Subtract1/2
  MinMax/1 -> Subtract2/1, Switch2/1
  Subtract2/1 -> CVサーボ時定数/1
  CVサーボ時定数/1 -> CVサーボ開閉時間/1
  CVサーボ開閉時間/1 -> 蒸気加減弁開度/1
  蒸気加減弁開度/1 -> 主蒸気流量/2, Subtract2/2, Cv/1
  高圧タービン/1 -> 中低圧タービン・再熱器/1, 高圧タービン分担比/1
  中低圧タービン・再熱器/1 -> 中低圧タービン分担比/1
  高圧タービン分担比/1 -> タービン出力/2
  中低圧タービン分担比/1 -> タービン出力/1
  タービン出力/1 -> 出力偏差/1, PG_CURRENT(pu)/1, 連続出力切替/1(モデル)
  GF・LL幅/1 -> Add2/1
  Add2/1 -> 追従回路/1(In)
  ボイラ特性/1 -> 主蒸気圧力 偏差/1
  圧力制御/1 -> 主蒸気圧力 偏差/2
  Subtract/1 -> ボイラ特性/1, 圧力制御/1
  出力上下限/1 -> ボイラ発生蒸気/1, MWDD/1, 出力制御遅れ/1, Switch3/3
  GF運転・LL運転/1 -> 負荷 設定/2, 負荷 制限/2, Switch2/2, Switch1/2
  負荷 設定/1 -> Subtract1/1, Pref/1
  追従回路/1(Out) -> 負荷 制限/1, 負荷 設定/3
  Switch2/1 -> Add2/2
  MW->pu/1 -> MWD/1, 出力変化率/1, 連続出力切替/3(MWD)
  Hz->pu/1 -> 速度調定率/1, 周波数バイアス/1
  連続出力切替/1(出力) -> pu->MW/1
  pu->MW/1 -> Mux5/2, タービン出力(MW)/1
  負荷 制限/1 -> MinMax/1, Ll/1
  周波数バイアス/1 -> Switch1/1
  Constant/1 -> Switch1/3
  Switch1/1 -> Add/1
  出力制御遅れ/1 -> Switch3/1
  Switch3/1 -> 出力偏差/2
  出力制御遅れ有無/1 -> Switch3/2
  EDC指令値(MW)/1 -> MWD(MW)/2, Mux5/1, 運転モード/1
  LFC指令値(MW)/1 -> MWD(MW)/1
  運転モード/1 -> 連続出力切替/2(運転モード)
  Mux5/1 -> Scope1/1

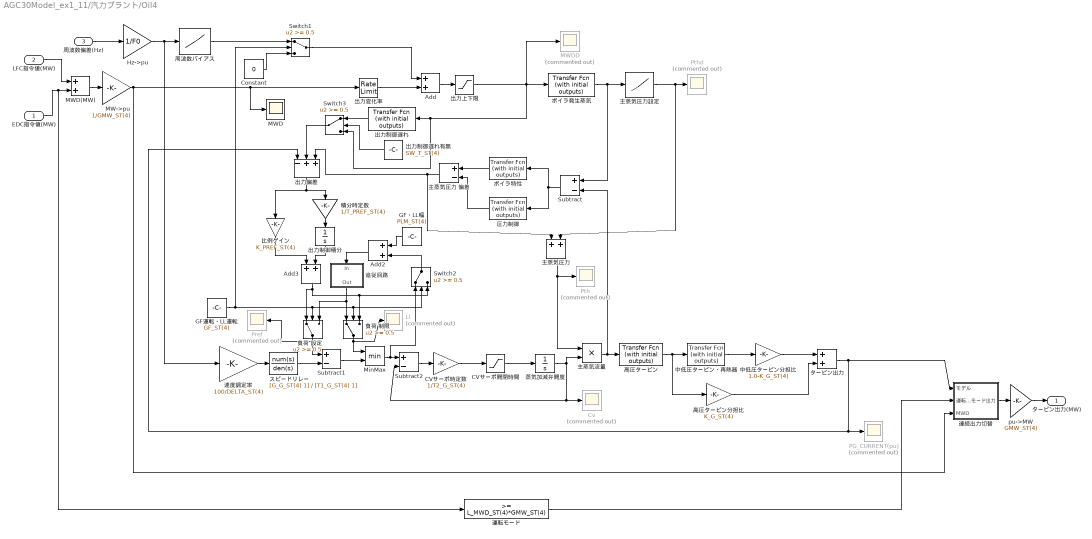
== system AGC30Model_ex1_11/汽力プラント/Oil4 ==
  EDC指令値(MW) : Inport
  LFC指令値(MW) : Inport  Port=2
  周波数偏差(Hz) : Inport  Port=3
  Add : Sum
  Add2 : Sum
  Add3 : Sum
  CVサーボ時定数 : Gain  Gain=1/T2_G_ST(4)
  CVサーボ開閉時間 : Saturate  UpperLimit=1/T3_G_ST(4)  LowerLimit=1/T6_G_ST(4)
  Constant : Constant  Value=0
  Cv : Scope  Commented=on
  GF・LL幅 : Constant  Value=PLM_ST(4)
  GF運転・LL運転 : Constant  Value=GF_ST(4)
  Hz->pu : Gain  Gain=1/F0
  Ll : Scope  Commented=on
  MW->pu : Gain  Gain=1/GMW_ST(4)
  MWD : Scope
  MWD(MW) : Sum
  MWDD : Scope  Commented=on
  MinMax : MinMax  Inputs=2
  PG_CURRENT(pu) : Scope  Commented=on
  Pref : Scope  Commented=on
  Pth : Scope  Commented=on
  Pthd : Scope  Commented=on
  Subtract : Sum  Inputs=+-
  Subtract1 : Sum  Inputs=+-
  Subtract2 : Sum  Inputs=+-
  Switch1 : Switch  Threshold=0.5
  Switch2 : Switch  Threshold=0.5
  Switch3 : Switch  Threshold=0.5
  pu->MW : Gain  Gain=GMW_ST(4)
  スピードリレー : TransferFcn  Numerator=[G_G_ST(4) 1]  Denominator=[T1_G_ST(4) 1]
  タービン出力 : Sum
  ボイラ特性 : simulink_extras/Additional Linear/Transfer Fcn (with initial outputs)  N=[1]  D=[T2_B_ST(4) 1]  Y0=0  U0=0
  ボイラ発生蒸気 : simulink_extras/Additional Linear/Transfer Fcn (with initial outputs)  N=[1]  D=[T1_B_ST(4) 1]  Y0=MW0_ST(4)  U0=MW0_ST(4)
  中低圧タービン・再熱器 : simulink_extras/Additional Linear/Transfer Fcn (with initial outputs)  N=[1]  D=[T5_G_ST(4) 1]  Y0=MW0_ST(4)  U0=MW0_ST(4)
  中低圧タービン分担比 : Gain  Gain=1.0-K_G_ST(4)
  主蒸気圧力 : Sum
  主蒸気圧力 偏差 : Sum  Inputs=+-
  主蒸気圧力設定 : Lookup  InputValues=FX_PTHD_ST(:,4)  Table=FY_PTHD_ST(:,4)  LookUpMeth=Interpolation-Use End Values
  主蒸気流量 : Product  RndMeth=Zero
  出力上下限 : Saturate  UpperLimit=U_MWD_ST(4)  LowerLimit=L_MWD_ST(4)
  出力偏差 : Sum  Inputs=-++
  出力制御積分 : Integrator  InitialCondition=MW0_ST(4)/PTH0_ST(4)  LimitOutput=on  UpperSaturationLimit=U_PREF_ST(4)  LowerSaturationLimit=L_PREF_ST(4)
  出力制御遅れ : simulink_extras/Additional Linear/Transfer Fcn (with initial outputs)  N=[1]  D=[T_T_ST(4) 1]  Y0=MW0_ST(4)  U0=MW0_ST(4)
  出力制御遅れ有無 : Constant  Value=SW_T_ST(4)
  出力変化率 : RateLimiter  RisingSlewLimit=R_MWD_ST(4)/60  FallingSlewLimit=-R_MWD_ST(4)/60  SampleTimeMode=inherited  InitialCondition=MW0_ST(4)
  周波数バイアス : Lookup  InputValues=FX_FB_ST(:,4)/F0  Table=FY_FB_ST(:,4)  LookUpMeth=Interpolation-Use End Values
  圧力制御 : simulink_extras/Additional Linear/Transfer Fcn (with initial outputs)  N=[1]  D=[T3_B_ST(4) 1]  Y0=0  U0=0
  比例ゲイン : Gain  Gain=K_PREF_ST(4)
  積分時定数 : Gain  Gain=1/T_PREF_ST(4)
  蒸気加減弁開度 : Integrator  InitialCondition=MW0_ST(4)/PTH0_ST(4)  LimitOutput=on  UpperSaturationLimit=U_G_ST(4)  LowerSaturationLimit=L_G_ST(4)
  負荷 制限 : Switch  Threshold=0.5
  負荷 設定 : Switch  Threshold=0.5
  追従回路 : Subsystem
  速度調定率 : Gain  Gain=100/DELTA_ST(4)
  連続出力切替 : Subsystem
  運転モード : simulink/Logic and Bit Operations/Compare To Constant  relop=>=  const=L_MWD_ST(4)*GMW_ST(4)  OutDataTypeStr=boolean
  高圧タービン : simulink_extras/Additional Linear/Transfer Fcn (with initial outputs)  N=[1]  D=[T4_G_ST(4) 1]  Y0=MW0_ST(4)  U0=MW0_ST(4)
  高圧タービン分担比 : Gain  Gain=K_G_ST(4)
  タービン出力(MW) : Outport  VectorParamsAs1DForOutWhenUnconnected=off
  wires:
  MWD(MW)/1 -> MW->pu/1
  周波数偏差(Hz)/1 -> Hz->pu/1
  Add/1 -> 出力上下限/1
  出力変化率/1 -> Add/2
  ボイラ発生蒸気/1 -> Subtract/1, 主蒸気圧力設定/1
  出力偏差/1 -> 比例ゲイン/1, 積分時定数/1
  比例ゲイン/1 -> Add3/1
  Add3/1 -> 負荷 制限/3, Switch2/3, 負荷 設定/1
  主蒸気圧力 偏差/1 -> 主蒸気圧力/1, 出力偏差/3
  主蒸気圧力設定/1 -> Pthd/1, 主蒸気圧力/2
  主蒸気流量/1 -> Subtract/2, 高圧タービン/1
  積分時定数/1 -> 出力制御積分/1
  出力制御積分/1 -> Add3/2
  速度調定率/1 -> スピードリレー/1
  Subtract1/1 -> MinMax/2
  主蒸気圧力/1 -> 主蒸気流量/1, Pth/1
  スピードリレー/1 -> Subtract1/2
  MinMax/1 -> Subtract2/1, Switch2/1
  Subtract2/1 -> CVサーボ時定数/1
  CVサーボ時定数/1 -> CVサーボ開閉時間/1
  CVサーボ開閉時間/1 -> 蒸気加減弁開度/1
  蒸気加減弁開度/1 -> 主蒸気流量/2, Subtract2/2, Cv/1
  高圧タービン/1 -> 中低圧タービン・再熱器/1, 高圧タービン分担比/1
  中低圧タービン・再熱器/1 -> 中低圧タービン分担比/1
  高圧タービン分担比/1 -> タービン出力/2
  中低圧タービン分担比/1 -> タービン出力/1
  タービン出力/1 -> 出力偏差/1, PG_CURRENT(pu)/1, 連続出力切替/1(モデル)
  GF・LL幅/1 -> Add2/1
  Add2/1 -> 追従回路/1(In)
  ボイラ特性/1 -> 主蒸気圧力 偏差/1
  圧力制御/1 -> 主蒸気圧力 偏差/2
  Subtract/1 -> ボイラ特性/1, 圧力制御/1
  出力上下限/1 -> ボイラ発生蒸気/1, MWDD/1, 出力制御遅れ/1, Switch3/3
  GF運転・LL運転/1 -> 負荷 設定/2, 負荷 制限/2, Switch2/2, Switch1/2
  負荷 設定/1 -> Subtract1/1, Pref/1
  追従回路/1(Out) -> 負荷 制限/1, 負荷 設定/3
  Switch2/1 -> Add2/2
  MW->pu/1 -> MWD/1, 出力変化率/1, 連続出力切替/3(MWD)
  Hz->pu/1 -> 速度調定率/1, 周波数バイアス/1
  連続出力切替/1(出力) -> pu->MW/1
  pu->MW/1 -> タービン出力(MW)/1
  負荷 制限/1 -> MinMax/1, Ll/1
  周波数バイアス/1 -> Switch1/1
  Constant/1 -> Switch1/3
  Switch1/1 -> Add/1
  出力制御遅れ/1 -> Switch3/1
  Switch3/1 -> 出力偏差/2
  出力制御遅れ有無/1 -> Switch3/2
  EDC指令値(MW)/1 -> MWD(MW)/2, 運転モード/1
  LFC指令値(MW)/1 -> MWD(MW)/1
  運転モード/1 -> 連続出力切替/2(運転モード)

== system AGC30Model_ex1_11/GTCCプラント/GTCC1/IGV制御 ==
  排ガス温度計測値 : Inport
  ガスタービン出力 : Inport  Port=2
  IGVアクチュエータ : simulink_extras/Additional Linear/Transfer Fcn (with initial outputs)  N=[1]  D=[T_IGVA_CC(1) 1]  Y0=IGV0_CC(1)  U0=IGV0_CC(1)
  IGV制御 : pid_lib/PID Controller  Controller=PI  Form=Parallel  TimeDomain=Continuous-time  UseExternalTs=off  SampleTime=-1  IntegratorMethod=Forward Euler  FilterMethod=Forward Euler  ControllerParametersSource=internal  P=K_IGV_CC(1)  I=1/T_IGV_CC(1)  D=0  UseFilter=on  N=0  TunerSelectOption=Transfer Function Based (PID Tuner App)  InitialConditionSource=internal  InitialConditionForIntegrator=IGV0_CC(1)  InitialConditionForFilter=0  DifferentiatorICPrevScaledInput=0  ExternalReset=none  TrackingMode=off  Kt=1  LimitOutput=on  SatLimitsSource=internal  UpperSaturationLimit=U_IGV_CC(1)  LowerSaturationLimit=L_IGV_CC(1)  LinearizeAsGain=off  AntiWindupMode=back-calculation  Kb=1/dtload  POutMin=[]  POutMax=[]  IOutMin=[]  IOutMax=[]  DOutMin=[]  DOutMax=[]  NOutMin=[]  NOutMax=[]  SumOutMin=[]  SumOutMax=[]  SaturationOutMin=[]  SaturationOutMax=[]  PParamMin=[]  PParamMax=[]  IParamMin=[]  IParamMax=[]  DParamMin=[]  DParamMax=[]  NParamMin=[]  NParamMax=[]  KbParamMin=[]  KbParamMax=[]  KtParamMin=[]  KtParamMax=[]  KbOutMin=[]  KbOutMax=[]  KtOutMin=[]  KtOutMax=[]  IntegratorOutMin=[]  IntegratorOutMax=[]  FilterOutMin=[]  FilterOutMax=[]  SumI1OutMin=[]  SumI1OutMax=[]  SumI2OutMin=[]  SumI2OutMax=[]  SumI3OutMin=[]  SumI3OutMax=[]  SumI4OutMin=[]  SumI4OutMax=[]  SumDOutMin=[]  SumDOutMax=[]  DifferentiatorOutMin=[]  DifferentiatorOutMax=[]  FilterDiffOutCoefMin=[]  FilterDiffOutCoefMax=[]  ReciprocalOutMin=[]  ReciprocalOutMax=[]  SumDenOutMin=[]  SumDenOutMax=[]  SumNumOutMin=[]  SumNumOutMax=[]  DivideOutMin=[]  DivideOutMax=[]  UdiffTsProdOutMin=[]  UdiffTsProdOutMax=[]  NTsProdOutMin=[]  NTsProdOutMax=[]  UintegralTsProdOutMin=[]  UintegralTsProdOutMax=[]  UngainTsProdOutMin=[]  UngainTsProdOutMax=[]  IntegratorContinuousStateAttributes=''  IntegratorStateMustResolveToSignalObject=off  IntegratorRTWStateStorageClass=Auto  FilterContinuousStateAttributes=''  FilterStateMustResolveToSignalObject=off  FilterRTWStateStorageClass=Auto  ParallelPVariant=InternalParameters  IdealPVariant=Disabled  IVariant=InternalParameters  DVariant=Disabled  IntegratorVariant=Continuous  SatVariant=Enabled  AWVariant=BackCalculation  PCopyVariant=Disabled  TRVariant=Disabled  FdbkBlocksVariant=Forward  IdealPFdbkVariant=Disabled  SatFdbkVariant=Disabled  DerivativeFilterVariant=Disabled  NVariant=Disabled  NCopyVariant=Disabled_SignalSpec  FilterICVariant=Disabled  IntegratorICVariant=InternalICs  ExternalResetVariant=Disabled  TRSumVariant=Passthrough  SumFdbkVariant=Disabled  SumVariant=Sum_PI  TsampFilterVariant=InternalTs  TsampNgainVariant=Passthrough  TsampIntegralVariant=Passthrough  ExternalSaturationOutDataTypeStr=Inherit: Same as second input
  ガスタービン定格出力ベース : Gain  Gain=1/FGT_CC(1)
  排ガス温度偏差 : Sum  Inputs=+-
  排ガス温度設定値 : Lookup  InputValues=FX_TE2_CC(:,1)  Table=FY_TE2_CC(:,1)  LookUpMeth=Interpolation-Use End Values
  IGV開度 : Outport  VectorParamsAs1DForOutWhenUnconnected=off
  wires:
  ガスタービン出力/1 -> ガスタービン定格出力ベース/1
  IGVアクチュエータ/1 -> IGV開度/1
  排ガス温度計測値/1 -> 排ガス温度偏差/1
  排ガス温度設定値/1 -> 排ガス温度偏差/2
  IGV制御/1 -> IGVアクチュエータ/1
  排ガス温度偏差/1 -> IGV制御/1
  ガスタービン定格出力ベース/1 -> 排ガス温度設定値/1

== system AGC30Model_ex1_11/GTCCプラント/GTCC1/ガスタービン ==
  燃料流量 : Inport
  周波数偏差 : Inport  Port=2
  IGV開度 : Inport  Port=3
  出力特性 : Subsystem
  温度特性 : Subsystem
  空気流量 : Subsystem
  ガスタービン出力 : Outport  VectorParamsAs1DForOutWhenUnconnected=off
  "空気流量 " : Outport  Port=2  VectorParamsAs1DForOutWhenUnconnected=off
  排ガス温度 : Outport  Port=3  VectorParamsAs1DForOutWhenUnconnected=off
  wires:
  燃料流量/1 -> 温度特性/1(燃料流量)
  温度特性/4(排ガス温度) -> 出力特性/4(排ガス温度), 排ガス温度/1
  温度特性/3(ガスタービン入口温度) -> 出力特性/3(ガスタービン入口温度)
  温度特性/2(圧縮機出口温度) -> 出力特性/2(圧縮機出口温度)
  出力特性/1(ガスタービン出力) -> ガスタービン出力/1
  温度特性/1(大気温度) -> 出力特性/1(大気温度)
  IGV開度/1 -> 空気流量/1(IGV開度)
  周波数偏差/1 -> 空気流量/2(周波数偏差)
  空気流量/1(空気流量) -> "空気流量 "/1, 出力特性/5(空気流量), 温度特性/2(空気流量)

== system AGC30Model_ex1_11/GTCCプラント/GTCC1/出力切替不連続防止 ==
  モデル : Inport
  運転モード : Inport  Port=2
  出力指令値 : Inport  Port=3
  Add : Sum
  Constant : Constant  Value=0
  Gain : Gain  Gain=-1
  Gain1 : Gain  Gain=-1
  Gain2 : Gain  Gain=-1
  MWD使用時に レートを制限 : Switch  Threshold=1
  MWD使用時はMWD-モデル モデル使用時は0 : Switch  Threshold=1
  MWD使用時はMWD-モデルに追従 モデル使用時はレートでMWD-モデルから0へ変化 （MWD⇒モデル時に不連続打消し分として使用） : simulink/Discontinuities/Rate Limiter Dynamic
  Subtract : Sum  Inputs=-+
  Switch1 : Switch  Threshold=1
  ∞ : Constant  Value=9999
  モデル使用時に レートを制限 : Switch  Threshold=1
  モデル使用時はモデル-MWD MWD使用時は0 : Switch  Threshold=1
  モデル使用時はモデル-MWDに追従 MWD使用時はレートでモデル-MWDから0に変化 （モデル⇒MWD時に不連続打消し分として使用） : simulink/Discontinuities/Rate Limiter Dynamic
  不連続 打消し分 : Switch  Threshold=1
  不連続分を 戻すレート : Constant  Value=0.0001
  出力 : Outport  VectorParamsAs1DForOutWhenUnconnected=off
  wires:
  出力指令値/1 -> Subtract/2, Switch1/3
  モデル/1 -> Switch1/1, Subtract/1
  Constant/1 -> MWD使用時はMWD-モデル モデル使用時は0/1, モデル使用時はモデル-MWD MWD使用時は0/3
  Subtract/1 -> Gain2/1, MWD使用時はMWD-モデル モデル使用時は0/3
  MWD使用時はMWD-モデル モデル使用時は0/1 -> MWD使用時はMWD-モデルに追従 モデル使用時はレートでMWD-モデルから0へ変化 （MWD⇒モデル時に不連続打消し分として使用）/2
  モデル使用時はモデル-MWD MWD使用時は0/1 -> モデル使用時はモデル-MWDに追従 MWD使用時はレートでモデル-MWDから0に変化 （モデル⇒MWD時に不連続打消し分として使用）/2
  モデル使用時はモデル-MWDに追従 MWD使用時はレートでモデル-MWDから0に変化 （モデル⇒MWD時に不連続打消し分として使用）/1 -> 不連続 打消し分/3
  MWD使用時はMWD-モデルに追従 モデル使用時はレートでMWD-モデルから0へ変化 （MWD⇒モデル時に不連続打消し分として使用）/1 -> 不連続 打消し分/1
  Add/1 -> 出力/1
  不連続分を 戻すレート/1 -> モデル使用時に レートを制限/1, MWD使用時に レートを制限/3
  ∞/1 -> モデル使用時に レートを制限/3, MWD使用時に レートを制限/1
  モデル使用時に レートを制限/1 -> MWD使用時はMWD-モデルに追従 モデル使用時はレートでMWD-モデルから0へ変化 （MWD⇒モデル時に不連続打消し分として使用）/1, Gain/1
  MWD使用時に レートを制限/1 -> モデル使用時はモデル-MWDに追従 MWD使用時はレートでモデル-MWDから0に変化 （モデル⇒MWD時に不連続打消し分として使用）/1, Gain1/1
  Gain/1 -> MWD使用時はMWD-モデルに追従 モデル使用時はレートでMWD-モデルから0へ変化 （MWD⇒モデル時に不連続打消し分として使用）/3
  Gain1/1 -> モデル使用時はモデル-MWDに追従 MWD使用時はレートでモデル-MWDから0に変化 （モデル⇒MWD時に不連続打消し分として使用）/3
  Gain2/1 -> モデル使用時はモデル-MWD MWD使用時は0/1
  Switch1/1 -> Add/1
  不連続 打消し分/1 -> Add/2
  運転モード/1 -> Switch1/2, MWD使用時はMWD-モデル モデル使用時は0/2, モデル使用時はモデル-MWD MWD使用時は0/2, モデル使用時に レートを制限/2, MWD使用時に レートを制限/2, 不連続 打消し分/2

== system AGC30Model_ex1_11/GTCCプラント/GTCC1/排ガス温度制御 ==
  燃料流量制御信号 : Inport
  排ガス温度 : Inport  Port=2
  ガスタービン出力 : Inport  Port=3
  Add : Sum
  ガスタービン定格出力ベース : Gain  Gain=1/FGT_CC(1)
  サーモカップル : simulink_extras/Additional Linear/Transfer Fcn (with initial outputs)  N=[1]  D=[T_TEM_CC(1) 1]  Y0=TE0_CC(1)  U0=TE0_CC(1)
  排ガス温度偏差 : Sum  Inputs=+-
  排ガス温度偏差ゲイン : Gain  Gain=K_TE_CC(1)
  排ガス温度制御一次遅れ : simulink_extras/Additional Linear/Transfer Fcn (with initial outputs)  N=[1]  D=[T_TE_CC(1) 1]  Y0=FFCS0_CC(1)  U0=FFCS0_CC(1)
  排ガス温度計測値換算係数 : Gain  Gain=1/TER_CC(1)
  排ガス温度設定値 : Lookup  InputValues=FX_TE1_CC(:,1)  Table=FY_TE1_CC(:,1)  LookUpMeth=Interpolation-Use End Values
  排ガス温度制御信号 : Outport  VectorParamsAs1DForOutWhenUnconnected=off
  排ガス温度計測値 : Outport  Port=2  VectorParamsAs1DForOutWhenUnconnected=off
  wires:
  ガスタービン出力/1 -> ガスタービン定格出力ベース/1
  排ガス温度設定値/1 -> 排ガス温度偏差/1
  燃料流量制御信号/1 -> 排ガス温度制御一次遅れ/1
  排ガス温度偏差/1 -> 排ガス温度偏差ゲイン/1
  排ガス温度制御一次遅れ/1 -> Add/1
  排ガス温度偏差ゲイン/1 -> Add/2
  Add/1 -> 排ガス温度制御信号/1
  排ガス温度/1 -> サーモカップル/1
  排ガス温度計測値換算係数/1 -> 排ガス温度計測値/1, 排ガス温度偏差/2
  ガスタービン定格出力ベース/1 -> 排ガス温度設定値/1
  サーモカップル/1 -> 排ガス温度計測値換算係数/1

== system AGC30Model_ex1_11/GTCCプラント/GTCC1/燃料制御 ==
  速度・負荷制御信号 : Inport
  負荷制限制御信号 : Inport  Port=2
  排ガス温度制御信号 : Inport  Port=3
  周波数偏差 : Inport  Port=4
  Product1 : Product  Inputs=3  RndMeth=Zero
  定格周波数[pu] : Constant
  最小値選択 : MinMax  Inputs=3
  無負荷時燃料流量 : Constant  Value=WF_MIN_CC(1)
  燃料制御信号上下限 : Saturate  UpperLimit=U_FUEL_CC(1)  LowerLimit=L_FUEL_CC(1)
  燃料流量指令 : Sum
  燃料系統 : simulink_extras/Additional Linear/Transfer Fcn (with initial outputs)  N=[1]  D=[T_FUEL_CC(1) 1]  Y0=WF0_CC(1)  U0=WF0_CC(1)
  燃料調整可能範囲 : Constant  Value=1-WF_MIN_CC(1)
  系統周波数[pu] : Sum
  燃料流量 : Outport  VectorParamsAs1DForOutWhenUnconnected=off
  燃料制御信号 : Outport  Port=2  VectorParamsAs1DForOutWhenUnconnected=off
  wires:
  燃料制御信号上下限/1 -> Product1/1
  燃料系統/1 -> 燃料流量/1
  燃料調整可能範囲/1 -> Product1/2
  Product1/1 -> 燃料流量指令/1
  無負荷時燃料流量/1 -> 燃料流量指令/2
  燃料流量指令/1 -> 燃料系統/1
  系統周波数[pu]/1 -> Product1/3
  定格周波数[pu]/1 -> 系統周波数[pu]/2
  周波数偏差/1 -> 系統周波数[pu]/1
  最小値選択/1 -> 燃料制御信号/1, 燃料制御信号上下限/1
  速度・負荷制御信号/1 -> 最小値選択/1
  負荷制限制御信号/1 -> 最小値選択/2
  排ガス温度制御信号/1 -> 最小値選択/3

== system AGC30Model_ex1_11/GTCCプラント/GTCC1/蒸気タービン ==
  空気流量 : Inport
  排ガス温度 : Inport  Port=2
  Product3 : Product  Inputs=3  RndMeth=Zero
  排熱回収ボイラ : simulink_extras/Additional Linear/Transfer Fcn (with initial outputs)  N=[1]  D=[T_B_CC(1) 1]  Y0=PMST0_CC(1)  U0=PMST0_CC(1)
  蒸気タービン出力係数 : Constant  Value=KST_CC(1)
  蒸気タービン出力 : Outport  VectorParamsAs1DForOutWhenUnconnected=off
  wires:
  排熱回収ボイラ/1 -> 蒸気タービン出力/1
  空気流量/1 -> Product3/2
  排ガス温度/1 -> Product3/1
  蒸気タービン出力係数/1 -> Product3/3
  Product3/1 -> 排熱回収ボイラ/1

== system AGC30Model_ex1_11/GTCCプラント/GTCC1/負荷制限制御 ==
  速度・負荷制御信号 : Inport
  燃料流量制御信号 : Inport  Port=2
  周波数偏差 : Inport  Port=3
  Add : Sum  Inputs=+++
  GF・LL幅 : Constant  Value=PLM_CC(1)
  GF運転・LL運転 : Constant  Value=GF_CC(1)
  LL運転・GF運転 : Gain  Gain=1-GF_CC(1)
  Switch : Switch  Criteria=u2 > Threshold
  負荷制限制御一次遅れ : simulink_extras/Additional Linear/Transfer Fcn (with initial outputs)  N=[1]  D=[T_LL_CC(1) 1]  Y0=FFCS0_CC(1)  U0=FFCS0_CC(1)
  速度調定率 : Gain  Gain=-100/DELTA_CC(1)
  負荷制限制御信号 : Outport  VectorParamsAs1DForOutWhenUnconnected=off
  wires:
  周波数偏差/1 -> LL運転・GF運転/1
  LL運転・GF運転/1 -> 速度調定率/1
  GF・LL幅/1 -> Add/1
  Add/1 -> 負荷制限制御信号/1
  燃料流量制御信号/1 -> 負荷制限制御一次遅れ/1
  負荷制限制御一次遅れ/1 -> Switch/1
  GF運転・LL運転/1 -> Switch/2
  速度・負荷制御信号/1 -> Switch/3
  Switch/1 -> Add/2
  速度調定率/1 -> Add/3

== system AGC30Model_ex1_11/GTCCプラント/GTCC1/速度・負荷制御 ==
  軸出力 : Inport
  出力指令値 : Inport  Port=2
  周波数偏差 : Inport  Port=3
  燃料流量制御信号 : Inport  Port=4
  排ガス温度制御信号 : Inport  Port=5
  Add : Sum  Inputs=-+
  Add1 : Sum
  GF運転・LL運転 : Gain  Gain=GF_CC(1)
  MinMax : MinMax  Inputs=2
  出力上下限 : Saturate  UpperLimit=U_MWD_CC(1)  LowerLimit=L_MWD_CC(1)
  出力偏差 : Sum  Inputs=-+
  出力変化率 : RateLimiter  RisingSlewLimit=R_MWD_CC(1)/60  FallingSlewLimit=-R_MWD_CC(1)/60  SampleTimeMode=inherited  InitialCondition=PG_INIT_CC(1)/GMW_CC(1)
  周波数バイアス : Lookup  InputValues=FX_FB_CC(:,1)/F0  Table=FY_FB_CC(:,1)  LookUpMeth=Interpolation-Use End Values
  変化率制限 : Saturate  UpperLimit=R_PREF_CC(1)/60  LowerLimit=-R_PREF_CC(1)/60
  排ガス温度制御モード 移行フラグ : Relay  OffSwitchValue=0
  補正後の出力指令値 MWD' : Sum
  負荷設定器 : Integrator  InitialCondition=FFCS0_CC(1)  LimitOutput=on  UpperSaturationLimit=U_PREF_CC(1)  LowerSaturationLimit=L_PREF_CC(1)
  負荷設定時定数 : Gain  Gain=1/T_PREF_CC(1)
  速度調定率 : Gain  Gain=-100/DELTA_CC(1)
  速度・負荷制御信号 : Outport  VectorParamsAs1DForOutWhenUnconnected=off
  wires:
  GF運転・LL運転/1 -> 周波数バイアス/1, 速度調定率/1
  出力指令値/1 -> 出力変化率/1
  周波数偏差/1 -> GF運転・LL運転/1
  出力変化率/1 -> 補正後の出力指令値 MWD'/1
  周波数バイアス/1 -> 補正後の出力指令値 MWD'/2
  補正後の出力指令値 MWD'/1 -> 出力上下限/1
  軸出力/1 -> 出力偏差/1
  出力上下限/1 -> 出力偏差/2
  出力偏差/1 -> 負荷設定時定数/1
  負荷設定器/1 -> Add1/1
  速度調定率/1 -> Add1/2
  Add1/1 -> 速度・負荷制御信号/1
  排ガス温度制御信号/1 -> Add/2
  Add/1 -> 排ガス温度制御モード 移行フラグ/1
  変化率制限/1 -> MinMax/2
  排ガス温度制御モード 移行フラグ/1 -> MinMax/1
  燃料流量制御信号/1 -> Add/1
  MinMax/1 -> 負荷設定器/1
  負荷設定時定数/1 -> 変化率制限/1

== system AGC30Model_ex1_11/他エリア発電プラント/他エリアモデル/追従回路 ==
  In : Inport
  Subtract2 : Sum  Inputs=+-
  追従回路積分 : Integrator  InitialCondition=1.0+PLM_B  UpperSaturationLimit=Inf  LowerSaturationLimit=0
  追従変化率 : Saturate  UpperLimit=R_LL_ST_OA(1)/60  LowerLimit=-R_LL_ST_OA(1)/60
  追従時定数 : Gain  Gain=1/T_LL_ST_OA(1)
  Out : Outport  VectorParamsAs1DForOutWhenUnconnected=off
  wires:
  Subtract2/1 -> 追従時定数/1
  追従時定数/1 -> 追従変化率/1
  追従変化率/1 -> 追従回路積分/1
  追従回路積分/1 -> Out/1, Subtract2/2
  In/1 -> Subtract2/1

== system AGC30Model_ex1_11/可変速揚水発電機/可変速揚水/揚水運転 ==
  In1 : Inport
  Action Port : ActionPort  ActionPortLabel=else
  "  ±1  " : Saturate  UpperLimit=1  LowerLimit=-1
  " ±1 " : Integrator  LimitOutput=on  UpperSaturationLimit=1  LowerSaturationLimit=-1
  0,1 : Saturate  UpperLimit=1  LowerLimit=0
  Sum1 : Sum  Inputs=+++
  Sum2 : Sum  Inputs=|+-
  Sum7 : Sum  Inputs=-+|
  Sum8 : Sum  Inputs=+-
  ±1 : Saturate  UpperLimit=1  LowerLimit=-1
  コンバータ : simulink_extras/Additional Linear/Transfer Fcn (with initial outputs)  N=[K1_CONV_VA(1)]  D="[T1_CONV_VA(1)  1]"  Y0=Y_PM_INIT_VA(1)  U0=Y_PM_INIT_VA(1)
  サーボモータ : simulink_extras/Additional Linear/Transfer Fcn (with initial outputs)  N=[K2_SERV_VA(1)]  D="[T3_SERV_VA(1)  T2_SERV_VA(1)  1]"  Y0=Y_PM_INIT_VA(1)  U0=Y_PM_INIT_VA(1)
  ポンプ特性 : Lookup_n-D  NumberOfTableDimensions=1  BreakpointsForDimension1=FX_T_PM_VA(:,1)  Table=FY_T_PM_VA(:,1)  RndMeth=Simplest  InputSameDT=on
  出力上下限 : Saturate  UpperLimit=U_MWD_PM_VA(1)  LowerLimit=L_MWD_PM_VA(1)
  励磁装置および発電電動機 : Subsystem
  回転子慣性 : simulink_extras/Additional Linear/Transfer Fcn (with initial outputs)  N=[1]  D="[M_VA(1)  0]"  Y0=N_PM_INIT_VA(1)  U0=0
  変化率リミッタ : RateLimiter  RisingSlewLimit=RATE_PM_VA(1)  FallingSlewLimit=-RATE_PM_VA(1)
  微分 （リセットフィルタ） : TransferFcn  Numerator="[TD_SG_PM_VA(1)  0]"  Denominator="[TD_SG_PM_VA(1)  1]"
  微分ゲイン : Gain  Gain=KD_SG_PM_VA(1)
  最適回転速度 関数発生器 : Lookup_n-D  NumberOfTableDimensions=1  BreakpointsForDimension1=FX_N_PM_VA(:,1)  Table=FY_N_PM_VA(:,1)  DiagnosticForOutOfRangeInput=Error  RndMeth=Simplest  InputSameDT=on
  最適案内羽根開度 関数発生器 : Lookup_n-D  NumberOfTableDimensions=1  BreakpointsForDimension1=FX_Y_PM_VA(:,1)  Table=FY_Y_PM_VA(:,1)  DiagnosticForOutOfRangeInput=Error  RndMeth=Simplest  InputSameDT=on
  比例ゲイン : Gain  Gain=KP_SG_PM_VA(1)
  積分ゲイン : Gain  Gain=KI_SG_PM_VA(1)
  速度指令時定数 : simulink_extras/Additional Linear/Transfer Fcn (with initial outputs)  N=[1]  D="[T_N_VA(1)  1]"  Y0=N_PM_INIT_VA(1)  U0=N_PM_INIT_VA(1)
  Out2 : Outport  VectorParamsAs1DForOutWhenUnconnected=off
  wires:
  Sum8/1 -> 回転子慣性/1
  回転子慣性/1 -> ポンプ特性/1, Sum7/1  "回転速度"
  出力上下限/1 -> 変化率リミッタ/1
  最適案内羽根開度 関数発生器/1 -> コンバータ/1  "開度指令"
  速度指令時定数/1 -> Sum7/2
  最適回転速度 関数発生器/1 -> 速度指令時定数/1  "速度指令"
  サーボモータ/1 -> 0,1/1
  0,1/1 -> ?  "開度"
  ポンプ特性/1 -> Sum8/2  "ポンプ入力"
  励磁装置および発電電動機/1(Out1) -> Out2/1, Sum8/1  "有効電力入力"
  変化率リミッタ/1 -> Sum2/1, 最適案内羽根開度 関数発生器/1, 最適回転速度 関数発生器/1
  In1/1 -> 出力上下限/1  "有効電力指令"
  Sum2/1 -> 励磁装置および発電電動機/1(In1)
  コンバータ/1 -> サーボモータ/1
  Sum1/1 -> [SG_OUT]
  比例ゲイン/1 -> ±1/1
  " ±1 "/1 -> Sum1/2
  積分ゲイン/1 -> " ±1 "/1
  微分ゲイン/1 -> 微分 （リセットフィルタ）/1
  Sum7/1 -> 比例ゲイン/1, 微分ゲイン/1, 積分ゲイン/1
  微分 （リセットフィルタ）/1 -> "  ±1  "/1
  "  ±1  "/1 -> Sum1/3
  ±1/1 -> Sum1/1
  [SG_OUT] -> Sum2/2

== system AGC30Model_ex1_11/可変速揚水発電機/可変速揚水/発電運転 ==
  In1 : Inport
  Action Port : ActionPort  ActionPortLabel=if(u1 >= 0)
  "  ±1  " : Saturate  UpperLimit=1  LowerLimit=-1
  " ±1 " : Integrator  LimitOutput=on  UpperSaturationLimit=1  LowerSaturationLimit=-1
  0,1 : Saturate  UpperLimit=1  LowerLimit=0
  Sum : Sum  Inputs=++|
  Sum1 : Sum  Inputs=+++
  Sum7 : Sum  Inputs=-+|
  Sum8 : Sum  Inputs=-+
  ±1 : Saturate  UpperLimit=1  LowerLimit=-1
  ガイドベーン開度 出力換算係数 : Gain  Gain=K_MW_GV_VA(1)
  コンバータ : simulink_extras/Additional Linear/Transfer Fcn (with initial outputs)  N=[K1_CONV_VA(1)]  D="[T1_CONV_VA(1)  1]"  Y0=Y_GN_INIT_VA(1)  U0=Y_GN_INIT_VA(1)
  サーボモータ : simulink_extras/Additional Linear/Transfer Fcn (with initial outputs)  N=[K2_SERV_VA(1)]  D="[T3_SERV_VA(1)  T2_SERV_VA(1)  1]"  Y0=Y_GN_INIT_VA(1)  U0=Y_GN_INIT_VA(1)
  出力上下限 : Saturate  UpperLimit=U_MWD_GN_VA(1)  LowerLimit=L_MWD_GN_VA(1)
  励磁装置および発電電動機 : Subsystem
  回転子慣性 : simulink_extras/Additional Linear/Transfer Fcn (with initial outputs)  N=[1]  D="[M_VA(1)  0]"  Y0=N_GN_INIT_VA(1)  U0=0
  変化率リミッタ : RateLimiter  RisingSlewLimit=RATE_GN_VA(1)  FallingSlewLimit=-RATE_GN_VA(1)
  微分 （リセットフィルタ） : TransferFcn  Numerator="[TD_SG_GN_VA(1)  0]"  Denominator="[TD_SG_GN_VA(1)  1]"
  微分ゲイン : Gain  Gain=KD_SG_GN_VA(1)
  最適回転速度 関数発生器 : Lookup_n-D  NumberOfTableDimensions=1  BreakpointsForDimension1=FX_N_GN_VA(:,1)  Table=FY_N_GN_VA(:,1)  DiagnosticForOutOfRangeInput=Error  RndMeth=Simplest  InputSameDT=on
  最適案内羽根開度 関数発生器 : Lookup_n-D  NumberOfTableDimensions=1  BreakpointsForDimension1=FX_Y_GN_VA(:,1)  Table=FY_Y_GN_VA(:,1)  DiagnosticForOutOfRangeInput=Error  RndMeth=Simplest  InputSameDT=on
  比例ゲイン : Gain  Gain=KP_SG_GN_VA(1)
  水路特性 Tw=1.959 : simulink_extras/Additional Linear/Transfer Fcn (with initial outputs)  N="[-TW_WAY_VA(1)  1]"  D=[TW_WAY_VA(1)/2 1]  Y0=Y_GN_INIT_VA(1)*K_MW_GV_VA(1)  U0=Y_GN_INIT_VA(1)*K_MW_GV_VA(1)
  積分ゲイン : Gain  Gain=KI_SG_GN_VA(1)
  速度指令時定数 : simulink_extras/Additional Linear/Transfer Fcn (with initial outputs)  N=[1]  D="[T_N_VA(1)  1]"  Y0=N_GN_INIT_VA(1)  U0=N_GN_INIT_VA(1)
  Out1 : Outport  VectorParamsAs1DForOutWhenUnconnected=off
  wires:
  比例ゲイン/1 -> ±1/1
  " ±1 "/1 -> Sum1/2
  積分ゲイン/1 -> " ±1 "/1
  出力上下限/1 -> 変化率リミッタ/1
  微分ゲイン/1 -> 微分 （リセットフィルタ）/1
  Sum7/1 -> 比例ゲイン/1, 微分ゲイン/1, 積分ゲイン/1
  最適案内羽根開度 関数発生器/1 -> Sum/2  "開度指令"
  速度指令時定数/1 -> Sum7/2
  最適回転速度 関数発生器/1 -> 速度指令時定数/1  "速度指令"
  サーボモータ/1 -> 0,1/1
  微分 （リセットフィルタ）/1 -> "  ±1  "/1
  "  ±1  "/1 -> Sum1/3
  0,1/1 -> ガイドベーン開度 出力換算係数/1  "開度"
  Sum/1 -> コンバータ/1
  コンバータ/1 -> サーボモータ/1
  ±1/1 -> Sum1/1
  Sum1/1 -> Sum/1
  水路特性 Tw=1.959/1 -> Sum8/2  "水車出力"
  励磁装置および発電電動機/1(Out1) -> Out1/1, Sum8/1  "有効電力出力"
  In1/1 -> 出力上下限/1  "有効電力指令"
  変化率リミッタ/1 -> 励磁装置および発電電動機/1(In1), 最適回転速度 関数発生器/1, 最適案内羽根開度 関数発生器/1
  Sum8/1 -> 回転子慣性/1
  回転子慣性/1 -> Sum7/1  "回転速度"
  ガイドベーン開度 出力換算係数/1 -> 水路特性 Tw=1.959/1
